simulink model "Sim3_GFo_L_Filter"  (R2018a)
settings: Solver=ode1  StartTime=0.0  StopTime=2.5  FixedStep=Time_Step  MaxStep=1e-4  RelTol=1e-3
undefined symbols (not defined in the file): Lg, Rg, Theta0, Time_Step, Ug, V0, VSC01_id0
libraries: powerlib x43, Control_Lib x9, simulink x8, powerlib_meascontrol x1
(part 2 of 3)

== system Sim3_GFo_L_Filter/VSC_pwm ==
  note: do not modify this part if you use the update loaflow script
  note: Common Inputs
  note: Power part
  note: Measurements and normalization
  note: Control part
  dE_set (pu) : Inport
  dP_set (pu) : Inport  Port=2
  1/Ib2 : Gain  Gain=1/Vb2
  1/Ib3 : Gain  Gain=1/Ib2
  Add : Sum
  Add1 : Sum
  Bridge_Model : Subsystem
  Bus01 : powerlib/Measurements/Three-Phase V-I Measurement  VoltageMeasurement=phase-to-ground  SetLabelV=off  LabelV=Vabc  Vpu=off  VpuLL=off  CurrentMeasurement=yes  SetLabelI=off  LabelI=Iabc  Ipu=off  Pbase=100e6  Vbase=500e3  OutputType=Complex  PhasorSimulation=off  PSBequivalent=0
  Control loops : Subsystem
  DC Voltage Source : powerlib/Electrical Sources/DC Voltage Source  Amplitude=Udcn  Measurements=Voltage
  Memory1 : Memory  InitialCondition=[Va0 Vb0 Vc0]
  Output_Transformer : powerlib/Elements/Three-Phase Transformer (Two Windings)  Winding1Connection=Yg  Winding2Connection=Yg  CoreType=Three single-phase transformers  SetSaturation=off  Hysteresis=off  DataFile='hysteresis'  SetInitialFlux=off  Measurements=None  UNITS=pu  NominalPower=[Sn , fb]  Winding1=[Un1 , Rt_pu/2 , Lt_pu/2]  Winding2=[Un2 , Rt_pu/2 , Lt_pu/2]  Rm=Rm_pu  Lm=Lm_pu  L0=0.5  Saturation=[ 0,0 ; 0.0024,1.2 ; 1.0,1.52 ]  InitialFluxes=[ 0.8 , -0.8 , 0.7 ]  BreakLoop=off  DiscreteSolver=Trapezoidal iterative  DataType=off  TransfoNumber=1
  Pinit : Constant  Value=P0
  Source_For_LF : powerlib/Electrical Sources/Three-Phase Source  Commented=on  InternalConnection=Yg  VoltagePhases=off  Voltage=(400000)*1.00064  PhaseAngle=0.38118  Voltage_phases=[25e3 25e3 25e3]/sqrt(3)  PhaseAngles_phases=[0 -120 +120]  Frequency=fb  NonIdealSource=off  SpecifyImpedance=off  Resistance=0  Inductance=0  ShortCircuitLevel=100e6  BaseVoltage=Un  XRratio=7  BusType=PQ  Pref=P0*Sb  Qref=Q0*Sb  Prefabc=[10e3, 10e3, 10e3]  Qrefabc=[0, 0, 0]  Qmin=-inf  Qmax=inf
  Vvsc_init : Constant  Value=Vvsc0
  mp3 : Gain  Gain=Vb1
  A : PMIOPort  Side=Right
  B : PMIOPort  Port=2  Side=Right
  C : PMIOPort  Port=3  Side=Right
  m : Outport  VectorParamsAs1DForOutWhenUnconnected=off
  wires:
  Add/1 -> Control loops/2(P_set)
  Control loops/2(m) -> m/1  "Control"
  mp3/1 -> Memory1/1
  1/Ib3/1 -> Control loops/4(ig_abc_pu)  "ig_pu"
  1/Ib2/1 -> Control loops/3(vg_abc_pu)  "vg_pu"
  [vg_meas] -> 1/Ib2/1
  Control loops/1(vm_abc_ref_pu) -> mp3/1
  Add1/1 -> Control loops/1(E_set)
  Memory1/1 -> Bridge_Model/1(Uref)
  dP_set (pu)/1 -> Add/1
  Pinit/1 -> Add/2
  Vvsc_init/1 -> Add1/2
  Bus01/1 -> [vg_meas]
  dE_set (pu)/1 -> Add1/1
  Bus01/2 -> [ig_meas]
  [ig_meas] -> 1/Ib3/1
  connections:
  DC Voltage Source/LConn1 -- Bridge_Model/LConn2
  Output_Transformer/RConn1 -- Bus01/LConn1
  Output_Transformer/RConn2 -- Bus01/LConn2
  DC Voltage Source/RConn1 -- Bridge_Model/LConn1
  Output_Transformer/RConn3 -- Bus01/LConn3
  Source_For_LF/RConn2 -- B/RConn1 -- Bus01/RConn2
  Bridge_Model/RConn1 -- Output_Transformer/LConn1
  Bridge_Model/RConn2 -- Output_Transformer/LConn2
  Bridge_Model/RConn3 -- Output_Transformer/LConn3
  Source_For_LF/RConn1 -- A/RConn1 -- Bus01/RConn1
  Source_For_LF/RConn3 -- C/RConn1 -- Bus01/RConn3

== system Sim3_GFo_L_Filter/Infinite_Grid/ pu P//Q computation ==
  v_abc_pu : Inport  PortDimensions=3
  i_abc_pu : Inport  Port=2  PortDimensions=3
  Demux : Demux  Outputs=3
      settings: DisplayOption=none
  Mux : Mux  Inputs=3
  Product1 : Product  InputSameDT=on  SaturateOnIntegerOverflow=on  OutDataTypeStr=Inherit: Same as first input
  Product3 : Product  InputSameDT=on  SaturateOnIntegerOverflow=on  OutDataTypeStr=Inherit: Same as first input
  Sum : Sum  Inputs=+-  InputSameDT=on  SaturateOnIntegerOverflow=on  OutDataTypeStr=Inherit: Same as first input
  Sum1 : Sum  Inputs=1  InputSameDT=on  SaturateOnIntegerOverflow=on  OutDataTypeStr=Inherit: Same as first input
  Sum4 : Sum  Inputs=1  InputSameDT=on  SaturateOnIntegerOverflow=on  OutDataTypeStr=Inherit: Same as first input
  Sum5 : Sum  Inputs=+-  InputSameDT=on  SaturateOnIntegerOverflow=on  OutDataTypeStr=Inherit: Same as first input
  Sum6 : Sum  Inputs=+-  InputSameDT=on  SaturateOnIntegerOverflow=on  OutDataTypeStr=Inherit: Same as first input
  pu->V : Gain  Gain=1/sqrt(3)  SaturateOnIntegerOverflow=on  OutDataTypeStr=Inherit: Same as input  ParamDataTypeStr=Inherit: Same as input
  pu->V1 : Gain  Gain=1/3  SaturateOnIntegerOverflow=on  OutDataTypeStr=Inherit: Same as input  ParamDataTypeStr=Inherit: Same as input
  pu->V2 : Gain  Gain=1/3  SaturateOnIntegerOverflow=on  OutDataTypeStr=Inherit: Same as input  ParamDataTypeStr=Inherit: Same as input
  p_u : Outport  VectorParamsAs1DForOutWhenUnconnected=off
  q_u : Outport  Port=2  VectorParamsAs1DForOutWhenUnconnected=off
  wires:
  pu->V/1 -> pu->V2/1  "Q"
  Mux/1 -> Product3/1
  Sum6/1 -> Mux/2
  Sum5/1 -> Mux/1
  Sum/1 -> Mux/3
  Demux/3 -> Sum6/1, Sum5/2
  Demux/2 -> Sum5/1, Sum/2
  Demux/1 -> Sum6/2, Sum/1
  Sum4/1 -> pu->V1/1
  i_abc_pu/1 -> Product3/2, Product1/2
  v_abc_pu/1 -> Demux/1, Product1/1
  Product1/1 -> Sum4/1
  Product3/1 -> Sum1/1
  Sum1/1 -> pu->V/1
  pu->V1/1 -> p_u/1
  pu->V2/1 -> q_u/1

== system Sim3_GFo_L_Filter/Infinite_Grid/CosSin ==
  Theta_rad : Inport
  Mux : Mux  Inputs=2
  Trigonometric Function : Trigonometry
  Trigonometric Function1 : Trigonometry  Operator=cos
  CosSinTheta : Outport  VectorParamsAs1DForOutWhenUnconnected=off
  wires:
  Trigonometric Function1/1 -> Mux/1
  Mux/1 -> CosSinTheta/1
  Trigonometric Function/1 -> Mux/2
  Theta_rad/1 -> Trigonometric Function1/1, Trigonometric Function/1

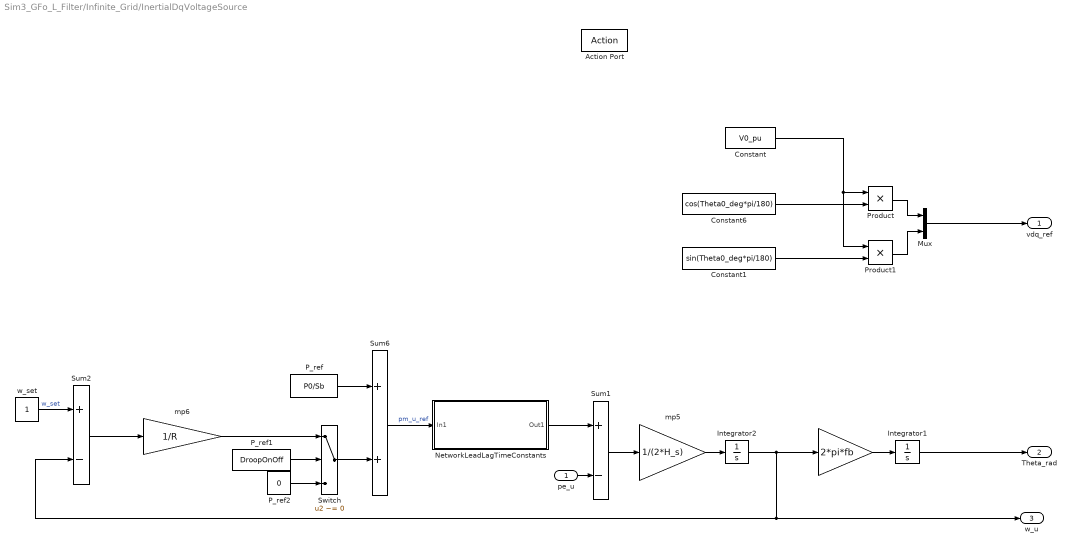
== system Sim3_GFo_L_Filter/Infinite_Grid/InertialDqVoltageSource ==
  pe_u : Inport
  Action Port : ActionPort
  " " : Gain  Gain=2*pi*fb
  Constant : Constant  Value=V0_pu
  Constant1 : Constant  Value=sin(Theta0_deg*pi/180)
  Constant6 : Constant  Value=cos(Theta0_deg*pi/180)
  Integrator1 : Integrator  InitialCondition=Theta0_deg*pi/180
  Integrator2 : Integrator  InitialCondition=1
  Mux : Mux  Inputs=2
  NetworkLeadLagTimeConstants : Subsystem
  P_ref : Constant  Value=P0/Sb
  P_ref1 : Constant  Value=DroopOnOff
  P_ref2 : Constant  Value=0
  Product : Product
  Product1 : Product
  Sum1 : Sum  Inputs=+-
  Sum2 : Sum  Inputs=+-
  Sum6 : Sum
  Switch : Switch  Criteria=u2 ~= 0
  mp5 : Gain  Gain=1/(2*H_s)
  mp6 : Gain  Gain=1/R
  w_set : Constant
  vdq_ref : Outport  VectorParamsAs1DForOutWhenUnconnected=off
  Theta_rad : Outport  Port=2  VectorParamsAs1DForOutWhenUnconnected=off
  w_u : Outport  Port=3  VectorParamsAs1DForOutWhenUnconnected=off
  wires:
  P_ref2/1 -> Switch/3
  mp6/1 -> Switch/1
  Switch/1 -> Sum6/2
  P_ref1/1 -> Switch/2
  NetworkLeadLagTimeConstants/1(Out1) -> Sum1/1
  Mux/1 -> vdq_ref/1
  Product/1 -> Mux/1
  Product1/1 -> Mux/2
  Constant/1 -> Product/1, Product1/1
  Constant6/1 -> Product/2
  Constant1/1 -> Product1/2
  Integrator1/1 -> Theta_rad/1
  w_set/1 -> Sum2/1  "w_set"
  pe_u/1 -> Sum1/2
  " "/1 -> Integrator1/1
  Sum1/1 -> mp5/1
  Sum2/1 -> mp6/1
  P_ref/1 -> Sum6/1
  Integrator2/1 -> " "/1, Sum2/2, w_u/1
  Sum6/1 -> NetworkLeadLagTimeConstants/1(In1)  "pm_u_ref"
  mp5/1 -> Integrator2/1

== system Sim3_GFo_L_Filter/Infinite_Grid/InfiniteDqVoltageSource ==
  Action Port : ActionPort
  Constant : Constant  Value=V0_pu
  Constant1 : Constant  Value=sin(Theta0_deg*pi/180)
  Constant4 : Constant
  Constant6 : Constant  Value=cos(Theta0_deg*pi/180)
  Gain : Gain  Gain=2*pi*fn
  Integrator : Integrator  InitialCondition=Theta0_deg*pi/180
  Mux : Mux  Inputs=2
  Product : Product
  Product1 : Product
  vdq_u_ref : Outport  VectorParamsAs1DForOutWhenUnconnected=off
  Theta_rad : Outport  Port=2  VectorParamsAs1DForOutWhenUnconnected=off
  w_u : Outport  Port=3  VectorParamsAs1DForOutWhenUnconnected=off
  wires:
  Constant4/1 -> Gain/1, w_u/1
  Mux/1 -> vdq_u_ref/1
  Integrator/1 -> Theta_rad/1
  Product1/1 -> Mux/2
  Constant/1 -> Product/1, Product1/1
  Constant6/1 -> Product/2
  Product/1 -> Mux/1
  Gain/1 -> Integrator/1
  Constant1/1 -> Product1/2

== system Sim3_GFo_L_Filter/Infinite_Grid/Source_For_OP ==
  v_abc_ref : Inport
  Controlled Voltage Source1 : powerlib/Electrical Sources/Controlled Voltage Source  Initialize=off  Source_Type=AC  Amplitude=V0*Ub*sqrt(2/3)*sin(Theta0)  Phase=(Theta0*180/pi)  Frequency=fb  Measurements=None
  Controlled Voltage Source2 : powerlib/Electrical Sources/Controlled Voltage Source  Initialize=off  Source_Type=AC  Amplitude=V0*Ub*sqrt(2/3)*sin(Theta0-2*pi/3)  Phase=(Theta0*180/pi)-120  Frequency=fb  Measurements=None
  Controlled Voltage Source3 : powerlib/Electrical Sources/Controlled Voltage Source  Initialize=off  Source_Type=AC  Amplitude=V0*Ub*sqrt(2/3)*sin(Theta0-4*pi/3)  Phase=(Theta0*180/pi)+120  Frequency=fb  Measurements=None
  Demux : Demux  Outputs=3
  Step : Step  Time=1e-9  SampleTime=0
  Subsystem3 : Subsystem
  Three-Phase Source1 : powerlib/Electrical Sources/Three-Phase Source  InternalConnection=Yn  VoltagePhases=off  Voltage=V0_pu*Ub  PhaseAngle=Theta0_deg  Voltage_phases=[25e3 25e3 25e3]/sqrt(3)  PhaseAngles_phases=[0 -120 +120]  Frequency=fb  NonIdealSource=off  SpecifyImpedance=off  Resistance=0.8929  Inductance=16.58e-3  ShortCircuitLevel=100e6  BaseVoltage=25e3  XRratio=7  BusType=swing  Pref=10e3  Qref=0  Prefabc=[10e3, 10e3, 10e3]  Qrefabc=[0, 0, 0]  Qmin=-inf  Qmax=inf
  A : PMIOPort  Side=Right
  B : PMIOPort  Port=2  Side=Right
  C : PMIOPort  Port=3  Side=Right
  N : PMIOPort  Port=4  Side=Left
  wires:
  Step/1 -> Subsystem3/1(switch)
  Demux/3 -> Controlled Voltage Source3/1
  Demux/1 -> Controlled Voltage Source1/1
  v_abc_ref/1 -> Demux/1
  Demux/2 -> Controlled Voltage Source2/1
  connections:
  Three-Phase Source1/RConn3 -- Subsystem3/LConn6
  Three-Phase Source1/RConn2 -- Subsystem3/LConn5
  Three-Phase Source1/RConn1 -- Subsystem3/LConn4
  Controlled Voltage Source3/RConn1 -- Subsystem3/LConn3
  Controlled Voltage Source2/RConn1 -- Subsystem3/LConn2
  Controlled Voltage Source1/RConn1 -- Subsystem3/LConn1
  Subsystem3/RConn3 -- C/RConn1
  Subsystem3/RConn2 -- B/RConn1
  Subsystem3/RConn1 -- A/RConn1
  Controlled Voltage Source1/LConn1 -- Controlled Voltage Source2/LConn1 -- N/RConn1 -- Three-Phase Source1/LConn1 -- Controlled Voltage Source3/LConn1

== system Sim3_GFo_L_Filter/VSC_average/Bridge_Model ==
  Uref : Inport
  Constant : Constant
  Memory : Memory
  NOT1 : Logic  Operator=NOT  IconShape=distinctive  AllPortsSameDT=off  OutDataTypeStr=boolean
  Saturation : Saturate  UpperLimit=1  LowerLimit=-1
  Three-Phase Breaker1 : powerlib/Elements/Three-Phase Breaker  InitialState=closed  SwitchA=on  SwitchB=on  SwitchC=on  SwitchTimes="[4/60  10/60]"  External=on  BreakerResistance=0.001  SnubberResistance=1e6  SnubberCapacitance=inf  Measurements=None
  Three-Phase Breaker2 : powerlib/Elements/Three-Phase Breaker  InitialState=open  SwitchA=on  SwitchB=on  SwitchC=on  SwitchTimes="[4/60  10/60]"  External=on  BreakerResistance=0.001  SnubberResistance=1e6  SnubberCapacitance=inf  Measurements=None
  Three-Phase Source : powerlib/Electrical Sources/Three-Phase Source  InternalConnection=Yg  VoltagePhases=off  Voltage=Vvsc0*Un1  PhaseAngle=Theta_vsc0  Voltage_phases=[25e3 25e3 25e3]/sqrt(3)  PhaseAngles_phases=[0 -120 +120]  Frequency=fb  NonIdealSource=off  SpecifyImpedance=off  Resistance=0  Inductance=0  ShortCircuitLevel=100e6  BaseVoltage=VSC01_Un1  XRratio=7  BusType=swing  Pref=0.3  Qref=0  Prefabc=[10e3, 10e3, 10e3]  Qrefabc=[0, 0, 0]  Qmin=-Inf  Qmax=Inf
  Universal Bridge : powerlib/Power Electronics/Universal Bridge  Arms=3  SnubberResistance=1e5  SnubberCapacitance=inf  Device=Average-model based VSC  Ron=1e-3  Lon=0  ForwardVoltages="[  0  0  ]"  ForwardVoltage=0  GTOparameters=[ 10e-6 , 20e-6 ]  IGBTparameters=[ 1e-6 , 2e-6 ]  Measurements=None  Measurements_2=None  converterType=Rectifier
  mp3 : Gain  Gain=2/Udcn
  PhA : PMIOPort  Side=Right
  PhB : PMIOPort  Port=2  Side=Right
  PhC : PMIOPort  Port=3  Side=Right
  Vdc+ : PMIOPort  Port=4  Side=Left
  Vdc- : PMIOPort  Port=5  Side=Left
  wires:
  Saturation/1 -> Universal Bridge/1
  Constant/1 -> Memory/1
  NOT1/1 -> Three-Phase Breaker1/1
  Memory/1 -> NOT1/1, Three-Phase Breaker2/1
  mp3/1 -> Saturation/1
  Uref/1 -> mp3/1
  connections:
  Three-Phase Breaker2/LConn1 -- Three-Phase Breaker1/LConn1 -- PhA/RConn1
  Three-Phase Breaker2/LConn2 -- Three-Phase Breaker1/LConn2 -- PhB/RConn1
  Three-Phase Breaker2/LConn3 -- Three-Phase Breaker1/LConn3 -- PhC/RConn1
  Three-Phase Breaker2/RConn1 -- Universal Bridge/LConn1
  Three-Phase Breaker2/RConn2 -- Universal Bridge/LConn2
  Three-Phase Breaker2/RConn3 -- Universal Bridge/LConn3
  Three-Phase Source/RConn1 -- Three-Phase Breaker1/RConn1
  Three-Phase Source/RConn2 -- Three-Phase Breaker1/RConn2
  Three-Phase Source/RConn3 -- Three-Phase Breaker1/RConn3
  Universal Bridge/RConn1 -- Vdc+/RConn1
  Universal Bridge/RConn2 -- Vdc-/RConn1

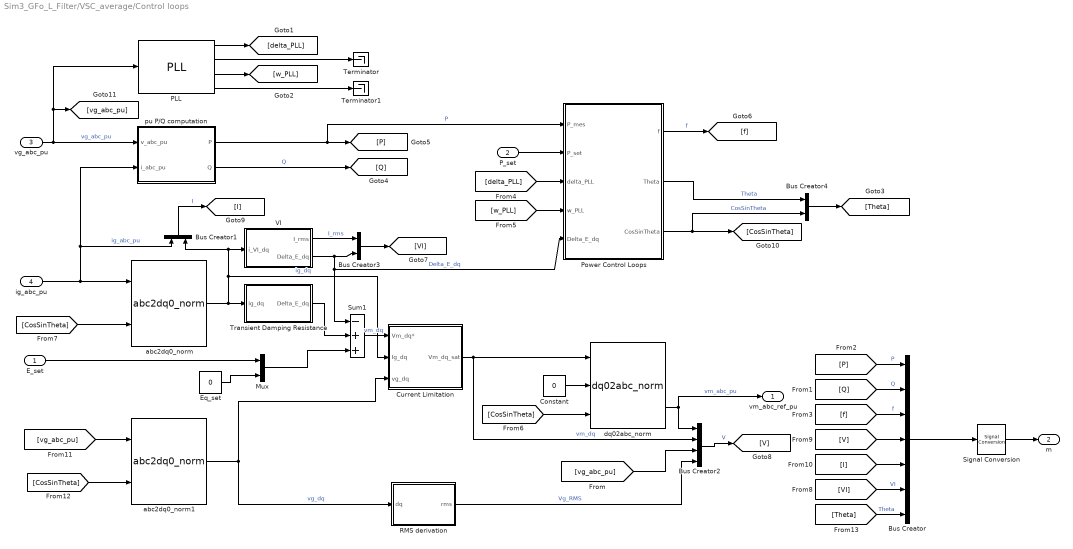
== system Sim3_GFo_L_Filter/VSC_average/Control loops ==
  E_set : Inport
  P_set : Inport  Port=2
  vg_abc_pu : Inport  Port=3
  ig_abc_pu : Inport  Port=4
  " pu P/Q computation" : Subsystem  DialogController=POWERSYS.PowerSysDialog
  Bus Creator : BusCreator  Inputs=7
  Bus Creator1 : BusCreator  Inputs=2
  Bus Creator2 : BusCreator  Inputs=4
  Bus Creator3 : BusCreator  Inputs=2
  Bus Creator4 : BusCreator  Inputs=2
  Constant : Constant  Value=0
  Current Limitation : Subsystem
  Eq_set : Constant  Value=0
  Mux : Mux  Inputs=2
  PLL : Control_Lib/PLL  fb=fb  Tr_PLL=Tr_PLL  Theta0=Theta0
      settings: SourceProductName=VSC_Lib
  Power Control Loops : Subsystem
  RMS derivation : Subsystem
  Signal Conversion : SignalConversion  OverrideOpt=off
  Sum1 : Sum  Inputs=-++
  Terminator : Terminator
  Terminator1 : Terminator
  Transient Damping Resistance : Subsystem
  VI : Subsystem
  abc2dq0_norm : Control_Lib/abc2dq0_norm  referenceAxisMode=Reference axis at 90 degrees behind phase_a  baseUpdateGain=1/sqrt(3)
      settings: SourceProductName=VSC_Lib
  abc2dq0_norm1 : Control_Lib/abc2dq0_norm  referenceAxisMode=Reference axis at 90 degrees behind phase_a  baseUpdateGain=1/sqrt(3)
      settings: SourceProductName=VSC_Lib
  dq02abc_norm : Control_Lib/dq02abc_norm  referenceAxisMode=Reference axis at 90 degrees behind phase_a  baseUpdateGain=sqrt(3)
      settings: SourceProductName=VSC_Lib
  vm_abc_ref_pu : Outport  VectorParamsAs1DForOutWhenUnconnected=off
  m : Outport  Port=2  VectorParamsAs1DForOutWhenUnconnected=off
  wires:
  [Theta] -> Bus Creator/7  "Theta"
  Bus Creator4/1 -> [Theta]
  RMS derivation/1(rms) -> Bus Creator2/4  "Vg_RMS"
  [vg_abc_pu] -> Bus Creator2/3
  Bus Creator3/1 -> [VI]
  PLL/4 -> Terminator1/1
  PLL/2 -> Terminator/1
  PLL/1 -> [delta_PLL]
  Constant/1 -> dq02abc_norm/2
  Power Control Loops/3(CosSinTheta) -> [CosSinTheta], Bus Creator4/2  "CosSinTheta"
  PLL/3 -> [w_PLL]
  [I] -> Bus Creator/5
  Bus Creator1/1 -> [I]  "I"
  Bus Creator/1 -> Signal Conversion/1
  [VI] -> Bus Creator/6  "VI"
  [V] -> Bus Creator/4
  Bus Creator2/1 -> [V]  "V"
  Eq_set/1 -> Mux/2
  Mux/1 -> Sum1/3
  VI/1(I_rms) -> Bus Creator3/1  "I_rms"
  Transient Damping Resistance/1("Delta_E_dq ") -> Sum1/2
  VI/2(Delta_E_dq) -> Bus Creator3/2, Sum1/1, Power Control Loops/5(Delta_E_dq)  "Delta_E_dq"
  [CosSinTheta] -> abc2dq0_norm/2
  [CosSinTheta] -> dq02abc_norm/3
  Power Control Loops/2(Theta) -> Bus Creator4/1  "Theta"
  abc2dq0_norm/2 -> Bus Creator1/2, VI/1(i_VI_dq), Current Limitation/2(Ig_dq), Transient Damping Resistance/1(ig_dq)  "ig_dq"
  ig_abc_pu/1 -> abc2dq0_norm/1, " pu P/Q computation"/2(i_abc_pu), Bus Creator1/1  "ig_abc_pu"
  " pu P/Q computation"/1(P) -> [P], Power Control Loops/1(P_mes)  "P"
  vg_abc_pu/1 -> PLL/1, [vg_abc_pu], " pu P/Q computation"/1(v_abc_pu)  "vg_abc_pu"
  Power Control Loops/1(f) -> [f]  "f"
  [w_PLL] -> Power Control Loops/4(w_PLL)
  P_set/1 -> Power Control Loops/2(P_set)
  [delta_PLL] -> Power Control Loops/3(delta_PLL)
  Current Limitation/1(Vm_dq_sat) -> dq02abc_norm/1, Bus Creator2/2  "vm_dq"
  " pu P/Q computation"/2(Q) -> [Q]  "Q"
  E_set/1 -> Mux/1
  dq02abc_norm/2 -> Bus Creator2/1, vm_abc_ref_pu/1  "vm_abc_pu"
  [f] -> Bus Creator/3  "f"
  [Q] -> Bus Creator/2  "Q"
  [P] -> Bus Creator/1  "P"
  Signal Conversion/1 -> m/1
  Sum1/1 -> Current Limitation/1(Vm_dq*)  "vm_dq"
  [vg_abc_pu] -> abc2dq0_norm1/1
  [CosSinTheta] -> abc2dq0_norm1/2
  abc2dq0_norm1/2 -> Current Limitation/3(vg_dq), RMS derivation/1(dq)  "vg_dq"

== system Sim3_GFo_L_Filter/VSC_pwm/Bridge_Model ==
  Uref : Inport
  Constant : Constant
  Detailed : Subsystem
  Memory : Memory
  NOT1 : Logic  Operator=NOT  IconShape=distinctive  AllPortsSameDT=off  OutDataTypeStr=boolean
  Saturation : Saturate  UpperLimit=1  LowerLimit=-1
  Three-Phase Breaker1 : powerlib/Elements/Three-Phase Breaker  InitialState=closed  SwitchA=on  SwitchB=on  SwitchC=on  SwitchTimes="[4/60  10/60]"  External=on  BreakerResistance=0.001  SnubberResistance=1e6  SnubberCapacitance=inf  Measurements=None
  Three-Phase Breaker2 : powerlib/Elements/Three-Phase Breaker  InitialState=open  SwitchA=on  SwitchB=on  SwitchC=on  SwitchTimes="[4/60  10/60]"  External=on  BreakerResistance=0.001  SnubberResistance=1e6  SnubberCapacitance=inf  Measurements=None
  Three-Phase Source : powerlib/Electrical Sources/Three-Phase Source  InternalConnection=Yg  VoltagePhases=off  Voltage=Vvsc0*Un1  PhaseAngle=Theta_vsc0  Voltage_phases=[25e3 25e3 25e3]/sqrt(3)  PhaseAngles_phases=[0 -120 +120]  Frequency=fb  NonIdealSource=off  SpecifyImpedance=off  Resistance=0  Inductance=0  ShortCircuitLevel=100e6  BaseVoltage=VSC01_Un1  XRratio=7  BusType=swing  Pref=0.3  Qref=0  Prefabc=[10e3, 10e3, 10e3]  Qrefabc=[0, 0, 0]  Qmin=-Inf  Qmax=Inf
  mp3 : Gain  Gain=2/Udcn
  PhA : PMIOPort  Side=Right
  PhB : PMIOPort  Port=2  Side=Right
  PhC : PMIOPort  Port=3  Side=Right
  Vdc+ : PMIOPort  Port=4  Side=Left
  Vdc- : PMIOPort  Port=5  Side=Left
  wires:
  Saturation/1 -> Detailed/1(Urref)
  Constant/1 -> Memory/1
  NOT1/1 -> Three-Phase Breaker1/1
  Memory/1 -> NOT1/1, Three-Phase Breaker2/1
  mp3/1 -> Saturation/1
  Uref/1 -> mp3/1
  connections:
  Three-Phase Breaker2/LConn1 -- Three-Phase Breaker1/LConn1 -- PhA/RConn1
  Three-Phase Breaker2/LConn2 -- Three-Phase Breaker1/LConn2 -- PhB/RConn1
  Three-Phase Breaker2/LConn3 -- Three-Phase Breaker1/LConn3 -- PhC/RConn1
  Detailed/LConn1 -- Three-Phase Breaker2/RConn1
  Detailed/LConn2 -- Three-Phase Breaker2/RConn2
  Detailed/LConn3 -- Three-Phase Breaker2/RConn3
  Three-Phase Source/RConn1 -- Three-Phase Breaker1/RConn1
  Three-Phase Source/RConn2 -- Three-Phase Breaker1/RConn2
  Three-Phase Source/RConn3 -- Three-Phase Breaker1/RConn3
  Detailed/RConn1 -- Vdc+/RConn1
  Detailed/RConn2 -- Vdc-/RConn1

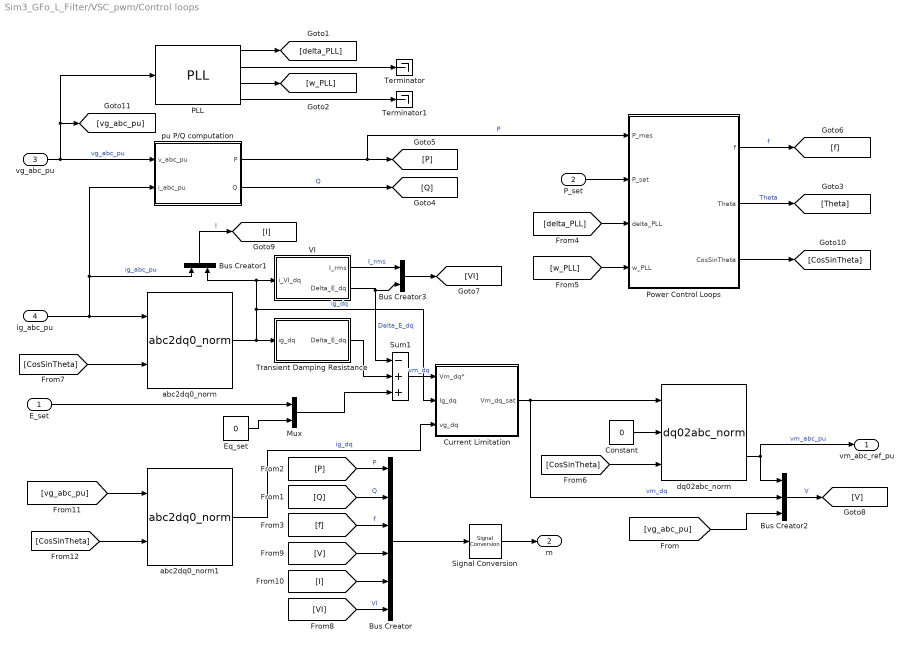
== system Sim3_GFo_L_Filter/VSC_pwm/Control loops ==
  E_set : Inport
  P_set : Inport  Port=2
  vg_abc_pu : Inport  Port=3
  ig_abc_pu : Inport  Port=4
  " pu P/Q computation" : Subsystem  DialogController=POWERSYS.PowerSysDialog
  Bus Creator : BusCreator  Inputs=6
  Bus Creator1 : BusCreator  Inputs=2
  Bus Creator2 : BusCreator  Inputs=3
  Bus Creator3 : BusCreator  Inputs=2
  Constant : Constant  Value=0
  Current Limitation : Subsystem
  Eq_set : Constant  Value=0
  Mux : Mux  Inputs=2
  PLL : Control_Lib/PLL  fb=fb  Tr_PLL=Tr_PLL  Theta0=Theta0
      settings: SourceProductName=VSC_Lib
  Power Control Loops : Subsystem
  Signal Conversion : SignalConversion  OverrideOpt=off
  Sum1 : Sum  Inputs=-++
  Terminator : Terminator
  Terminator1 : Terminator
  Transient Damping Resistance : Subsystem
  VI : Subsystem
  abc2dq0_norm : Control_Lib/abc2dq0_norm  referenceAxisMode=Reference axis at 90 degrees behind phase_a  baseUpdateGain=1/sqrt(3)
      settings: SourceProductName=VSC_Lib
  abc2dq0_norm1 : Control_Lib/abc2dq0_norm  referenceAxisMode=Reference axis at 90 degrees behind phase_a  baseUpdateGain=1/sqrt(3)
      settings: SourceProductName=VSC_Lib
  dq02abc_norm : Control_Lib/dq02abc_norm  referenceAxisMode=Reference axis at 90 degrees behind phase_a  baseUpdateGain=sqrt(3)
      settings: SourceProductName=VSC_Lib
  vm_abc_ref_pu : Outport  VectorParamsAs1DForOutWhenUnconnected=off
  m : Outport  Port=2  VectorParamsAs1DForOutWhenUnconnected=off
  wires:
  [vg_abc_pu] -> Bus Creator2/3
  Bus Creator3/1 -> [VI]
  PLL/4 -> Terminator1/1
  PLL/2 -> Terminator/1
  PLL/1 -> [delta_PLL]
  Constant/1 -> dq02abc_norm/2
  Power Control Loops/3(CosSinTheta) -> [CosSinTheta]
  PLL/3 -> [w_PLL]
  [I] -> Bus Creator/5
  Bus Creator1/1 -> [I]  "I"
  Bus Creator/1 -> Signal Conversion/1
  [VI] -> Bus Creator/6  "VI"
  [V] -> Bus Creator/4
  Bus Creator2/1 -> [V]  "V"
  Eq_set/1 -> Mux/2
  Mux/1 -> Sum1/3
  VI/1(I_rms) -> Bus Creator3/1  "I_rms"
  Transient Damping Resistance/1("Delta_E_dq ") -> Sum1/2
  VI/2(Delta_E_dq) -> Sum1/1, Bus Creator3/2  "Delta_E_dq"
  [CosSinTheta] -> abc2dq0_norm/2
  [CosSinTheta] -> dq02abc_norm/3
  Power Control Loops/2(Theta) -> [Theta]  "Theta"
  abc2dq0_norm/2 -> Bus Creator1/2, VI/1(i_VI_dq), Current Limitation/2(Ig_dq), Transient Damping Resistance/1(ig_dq)  "ig_dq"
  ig_abc_pu/1 -> abc2dq0_norm/1, " pu P/Q computation"/2(i_abc_pu), Bus Creator1/1  "ig_abc_pu"
  " pu P/Q computation"/1(P) -> [P], Power Control Loops/1(P_mes)  "P"
  vg_abc_pu/1 -> PLL/1, [vg_abc_pu], " pu P/Q computation"/1(v_abc_pu)  "vg_abc_pu"
  Power Control Loops/1(f) -> [f]  "f"
  [w_PLL] -> Power Control Loops/4(w_PLL)
  P_set/1 -> Power Control Loops/2(P_set)
  [delta_PLL] -> Power Control Loops/3(delta_PLL)
  Current Limitation/1(Vm_dq_sat) -> dq02abc_norm/1, Bus Creator2/2  "vm_dq"
  " pu P/Q computation"/2(Q) -> [Q]  "Q"
  E_set/1 -> Mux/1
  dq02abc_norm/2 -> Bus Creator2/1, vm_abc_ref_pu/1  "vm_abc_pu"
  [f] -> Bus Creator/3  "f"
  [Q] -> Bus Creator/2  "Q"
  [P] -> Bus Creator/1  "P"
  Signal Conversion/1 -> m/1
  Sum1/1 -> Current Limitation/1(Vm_dq*)  "vm_dq"
  [vg_abc_pu] -> abc2dq0_norm1/1
  [CosSinTheta] -> abc2dq0_norm1/2
  abc2dq0_norm1/2 -> Current Limitation/3(vg_dq)  "ig_dq"

== system Sim3_GFo_L_Filter/Infinite_Grid/InertialDqVoltageSource/NetworkLeadLagTimeConstants ==
  In1 : Inport
  Integrator3 : Integrator  InitialCondition=(P0/Sb)*(1-TN/TD)
  Sum1 : Sum
  Sum2 : Sum  Inputs=+-
  mp1 : Gain  Gain=TN/TD
  mp2 : Gain  Gain=1-TN/TD
  mp3 : Gain  Gain=1/TD
  Out1 : Outport  VectorParamsAs1DForOutWhenUnconnected=off
  wires:
  Sum2/1 -> mp3/1
  mp3/1 -> Integrator3/1
  Integrator3/1 -> Sum1/2, Sum2/2
  In1/1 -> mp1/1, mp2/1
  mp2/1 -> Sum2/1
  mp1/1 -> Sum1/1
  Sum1/1 -> Out1/1

== system Sim3_GFo_L_Filter/Infinite_Grid/Source_For_OP/Subsystem3 ==
  switch : Inport
  Breaker : powerlib/Elements/Breaker  InitialState=0  SwitchingTimes="[1/60  5/60]"  External=on  BreakerResistance=0.001  SnubberResistance=1e6  SnubberCapacitance=inf  Measurements=None  MoreParameters=on  NoBreakLoop=off
  Breaker1 : powerlib/Elements/Breaker  InitialState=0  SwitchingTimes="[1/60  5/60]"  External=on  BreakerResistance=0.001  SnubberResistance=1e6  SnubberCapacitance=inf  Measurements=None  MoreParameters=on  NoBreakLoop=off
  Breaker2 : powerlib/Elements/Breaker  InitialState=0  SwitchingTimes="[1/60  5/60]"  External=on  BreakerResistance=0.001  SnubberResistance=1e6  SnubberCapacitance=inf  Measurements=None  MoreParameters=on  NoBreakLoop=off
  Breaker3 : powerlib/Elements/Breaker  InitialState=1  SwitchingTimes="[1/60  5/60]"  External=on  BreakerResistance=0.001  SnubberResistance=1e6  SnubberCapacitance=inf  Measurements=None  MoreParameters=on  NoBreakLoop=off
  Breaker4 : powerlib/Elements/Breaker  InitialState=1  SwitchingTimes="[1/60  5/60]"  External=on  BreakerResistance=0.001  SnubberResistance=1e6  SnubberCapacitance=inf  Measurements=None  MoreParameters=on  NoBreakLoop=off
  Breaker5 : powerlib/Elements/Breaker  InitialState=1  SwitchingTimes="[1/60  5/60]"  External=on  BreakerResistance=0.001  SnubberResistance=1e6  SnubberCapacitance=inf  Measurements=None  MoreParameters=on  NoBreakLoop=off
  Logical Operator : Logic  Operator=NOT  AllPortsSameDT=off  OutDataTypeStr=boolean
  A : PMIOPort  Side=Left
  B : PMIOPort  Port=2  Side=Left
  C : PMIOPort  Port=3  Side=Left
  Ainit : PMIOPort  Port=4  Side=Left
  Binit : PMIOPort  Port=5  Side=Left
  Cinit : PMIOPort  Port=6  Side=Left
  a : PMIOPort  Port=7  Side=Right
  b : PMIOPort  Port=8  Side=Right
  c : PMIOPort  Port=9  Side=Right
  wires:
  Logical Operator/1 -> Breaker3/1, Breaker4/1, Breaker5/1
  switch/1 -> Logical Operator/1, Breaker/1, Breaker1/1, Breaker2/1
  connections:
  Breaker4/RConn1 -- Breaker1/RConn1 -- b/RConn1
  a/RConn1 -- Breaker3/RConn1 -- Breaker/RConn1
  Breaker1/LConn1 -- B/RConn1
  Breaker3/LConn1 -- Ainit/RConn1
  Breaker2/LConn1 -- C/RConn1
  Breaker4/LConn1 -- Binit/RConn1
  Breaker2/RConn1 -- Breaker5/RConn1 -- c/RConn1
  Breaker5/LConn1 -- Cinit/RConn1
  Breaker/LConn1 -- A/RConn1

== system Sim3_GFo_L_Filter/VSC_average/Control loops/ pu P//Q computation ==
  v_abc_pu : Inport  PortDimensions=3
  i_abc_pu : Inport  Port=2  PortDimensions=3
  Demux : Demux  Outputs=3
      settings: DisplayOption=none
  Mux : Mux  Inputs=3
  Product1 : Product  InputSameDT=on  SaturateOnIntegerOverflow=on  OutDataTypeStr=Inherit: Same as first input
  Product3 : Product  InputSameDT=on  SaturateOnIntegerOverflow=on  OutDataTypeStr=Inherit: Same as first input
  Sum : Sum  Inputs=+-  InputSameDT=on  SaturateOnIntegerOverflow=on  OutDataTypeStr=Inherit: Same as first input
  Sum1 : Sum  Inputs=1  InputSameDT=on  SaturateOnIntegerOverflow=on  OutDataTypeStr=Inherit: Same as first input
  Sum4 : Sum  Inputs=1  InputSameDT=on  SaturateOnIntegerOverflow=on  OutDataTypeStr=Inherit: Same as first input
  Sum5 : Sum  Inputs=+-  InputSameDT=on  SaturateOnIntegerOverflow=on  OutDataTypeStr=Inherit: Same as first input
  Sum6 : Sum  Inputs=+-  InputSameDT=on  SaturateOnIntegerOverflow=on  OutDataTypeStr=Inherit: Same as first input
  pu->V : Gain  Gain=1/sqrt(3)  SaturateOnIntegerOverflow=on  OutDataTypeStr=Inherit: Same as input  ParamDataTypeStr=Inherit: Same as input
  pu->V1 : Gain  Gain=1/3  SaturateOnIntegerOverflow=on  OutDataTypeStr=Inherit: Same as input  ParamDataTypeStr=Inherit: Same as input
  pu->V2 : Gain  Gain=1/3  SaturateOnIntegerOverflow=on  OutDataTypeStr=Inherit: Same as input  ParamDataTypeStr=Inherit: Same as input
  P : Outport  VectorParamsAs1DForOutWhenUnconnected=off
  Q : Outport  Port=2  VectorParamsAs1DForOutWhenUnconnected=off
  wires:
  pu->V2/1 -> Q/1
  pu->V1/1 -> P/1
  Sum1/1 -> pu->V/1
  Product3/1 -> Sum1/1
  Product1/1 -> Sum4/1
  v_abc_pu/1 -> Product1/1, Demux/1
  i_abc_pu/1 -> Product1/2, Product3/2
  Sum4/1 -> pu->V1/1
  Demux/1 -> Sum/1, Sum6/2
  Demux/2 -> Sum/2, Sum5/1
  Demux/3 -> Sum5/2, Sum6/1
  Sum/1 -> Mux/3
  Sum5/1 -> Mux/1
  Sum6/1 -> Mux/2
  Mux/1 -> Product3/1
  pu->V/1 -> pu->V2/1  "Q"

== system Sim3_GFo_L_Filter/VSC_average/Control loops/Current Limitation ==
  note: Current limitation
  Vm_dq* : Inport
  Ig_dq : Inport  Port=2
  vg_dq : Inport  Port=3
  Constant : Constant  Value=I_max_pu
  Current control : Subsystem
  Demux : Demux  Outputs=2
  Demux2 : Demux  Outputs=2
  Inverse Current control : Subsystem
  Mux : Mux  Inputs=2
  Product{,1..3} (4 alike) : Product
  Saturation Dynamic : simulink/Discontinuities/Saturation Dynamic  OutMin=[]  OutMax=[]  OutDataTypeStr=Inherit: Same as second input  OutDataType=fixdt(1, 16)  OutScaling=2^-10  DoSatur=off
  Sqrt : Sqrt  SaturateOnIntegerOverflow=on
  Sum : Sum
  Trigonometric Function : Trigonometry  Operator=atan2  NumberOfIterations=5  OutputSignalType=real
  Trigonometric Function1 : Trigonometry  Operator=cos
  Trigonometric Function2 : Trigonometry
  w_set1 : Constant
  w_set2 : Constant
  w_set3 : Constant  Value=0
  Vm_dq_sat : Outport  VectorParamsAs1DForOutWhenUnconnected=off
  wires:
  w_set3/1 -> Saturation Dynamic/3
  Constant/1 -> Saturation Dynamic/1
  Mux/1 -> Current control/1(Ig_dq0*)
  Product/1 -> Mux/1
  Demux/1 -> Product1/1, Product1/2
  Demux/2 -> Product2/1, Product2/2
  Trigonometric Function2/1 -> Product3/2
  Product2/1 -> Sum/2
  Trigonometric Function1/1 -> Product/2
  Demux2/1 -> Trigonometric Function/2
  Trigonometric Function/1 -> Trigonometric Function2/1, Trigonometric Function1/1
  Saturation Dynamic/1 -> Product/1, Product3/1
  Product1/1 -> Sum/1
  Sqrt/1 -> Saturation Dynamic/2
  Demux2/2 -> Trigonometric Function/1
  Inverse Current control/1(Is_dq*) -> Demux2/1, Demux/1
  Sum/1 -> Sqrt/1
  Product3/1 -> Mux/2
  Ig_dq/1 -> Inverse Current control/2(Ig_dq), Current control/2(Ig_dq0)
  w_set1/1 -> Inverse Current control/4(w)
  w_set2/1 -> Current control/4(w)
  vg_dq/1 -> Current control/3(vg_dq0), Inverse Current control/3(vg_dq)
  Vm_dq*/1 -> Inverse Current control/1(Vm_dq*)
  Current control/1(vm) -> Vm_dq_sat/1

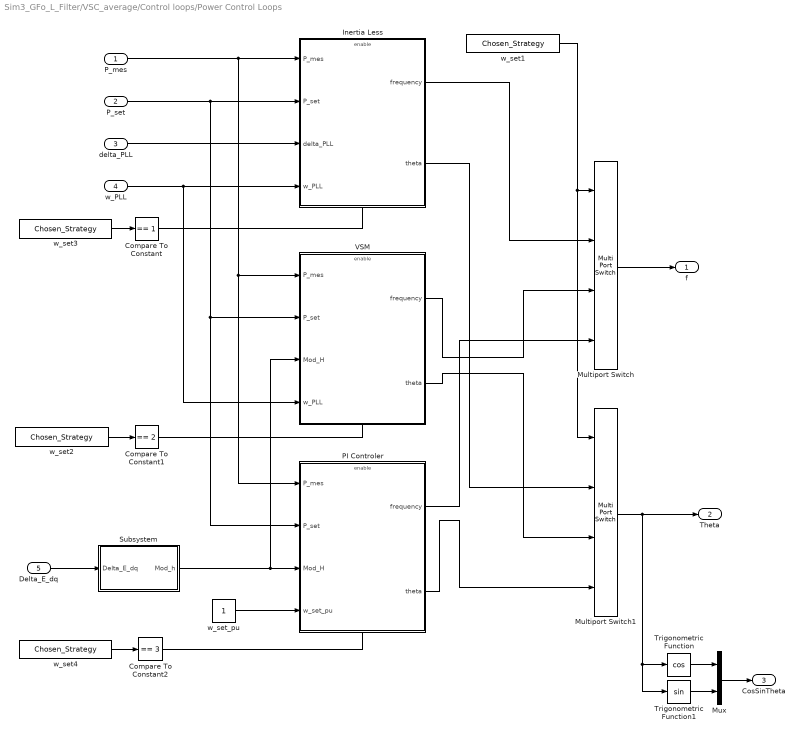
== system Sim3_GFo_L_Filter/VSC_average/Control loops/Power Control Loops ==
  P_mes : Inport
  P_set : Inport  Port=2
  delta_PLL : Inport  Port=3
  w_PLL : Inport  Port=4
  Delta_E_dq : Inport  Port=5
  Compare To Constant : simulink/Logic and Bit Operations/Compare To Constant  relop===  const=1  OutDataTypeStr=boolean
  Compare To Constant1 : simulink/Logic and Bit Operations/Compare To Constant  relop===  const=2  OutDataTypeStr=boolean
  Compare To Constant2 : simulink/Logic and Bit Operations/Compare To Constant  relop===  const=3  OutDataTypeStr=boolean
  Inertia Less : Subsystem
  Multiport Switch : MultiPortSwitch
  Multiport Switch1 : MultiPortSwitch
  Mux : Mux  Inputs=[1 1]
  PI Controler : Subsystem
  Subsystem : Subsystem
  Trigonometric Function : Trigonometry  Operator=cos
  Trigonometric Function1 : Trigonometry
  VSM : Subsystem
  w_set{1..4} (4 alike) : Constant  Value=Chosen_Strategy
  w_set_pu : Constant
  f : Outport  PortDimensions=1  VectorParamsAs1DForOutWhenUnconnected=off
  Theta : Outport  Port=2  VectorParamsAs1DForOutWhenUnconnected=off
  CosSinTheta : Outport  Port=3  PortDimensions=2  VectorParamsAs1DForOutWhenUnconnected=off
  wires:
  Subsystem/1(Mod_h) -> PI Controler/3(Mod_H), VSM/3(Mod_H)
  Delta_E_dq/1 -> Subsystem/1(Delta_E_dq)
  Multiport Switch1/1 -> Trigonometric Function1/1, Trigonometric Function/1, Theta/1
  Trigonometric Function1/1 -> Mux/2
  Mux/1 -> CosSinTheta/1
  Trigonometric Function/1 -> Mux/1
  Compare To Constant2/1 -> PI Controler/Enable
  Compare To Constant1/1 -> VSM/Enable
  Compare To Constant/1 -> Inertia Less/Enable
  w_set4/1 -> Compare To Constant2/1
  w_set2/1 -> Compare To Constant1/1
  w_set3/1 -> Compare To Constant/1
  Inertia Less/1(frequency) -> Multiport Switch/2
  Multiport Switch/1 -> f/1
  Inertia Less/2(theta) -> Multiport Switch1/2
  VSM/2(theta) -> Multiport Switch1/3
  w_set1/1 -> Multiport Switch/1, Multiport Switch1/1
  VSM/1(frequency) -> Multiport Switch/3
  PI Controler/1(frequency) -> Multiport Switch/4
  PI Controler/2(theta) -> Multiport Switch1/4
  w_set_pu/1 -> PI Controler/4(w_set_pu)
  w_PLL/1 -> Inertia Less/4(w_PLL), VSM/4(w_PLL)
  delta_PLL/1 -> Inertia Less/3(delta_PLL)
  P_set/1 -> Inertia Less/2(P_set), VSM/2(P_set), PI Controler/2(P_set)
  P_mes/1 -> Inertia Less/1(P_mes), VSM/1(P_mes), PI Controler/1(P_mes)

== system Sim3_GFo_L_Filter/VSC_average/Control loops/RMS derivation ==
  dq : Inport
  Demux : Demux  Outputs=2
  Sqrt : Sqrt  SaturateOnIntegerOverflow=on
  Square : Math  Operator=square  SaturateOnIntegerOverflow=on
  Square1 : Math  Operator=square  SaturateOnIntegerOverflow=on
  Sum : Sum
  rms : Outport
  wires:
  dq/1 -> Demux/1
  Demux/2 -> Square1/1
  Square/1 -> Sum/1
  Demux/1 -> Square/1
  Sqrt/1 -> rms/1
  Sum/1 -> Sqrt/1
  Square1/1 -> Sum/2

== system Sim3_GFo_L_Filter/VSC_average/Control loops/Transient Damping Resistance ==
  ig_dq : Inport
  Filter w_LF : Subsystem
      mask Display: disp('\omega_{LF} / (s + \omega_{LF})','texmode','on')
  Sum5 : Sum  Inputs=|+-
  nq1 : Gain  Gain=Rv
  "Delta_E_dq " : Outport  VectorParamsAs1DForOutWhenUnconnected=off
  wires:
  nq1/1 -> Filter w_LF/1(e), Sum5/2
  Filter w_LF/1(s) -> Sum5/1
  Sum5/1 -> "Delta_E_dq "/1
  ig_dq/1 -> nq1/1

== system Sim3_GFo_L_Filter/VSC_average/Control loops/VI ==
  note: VI triggering and threshold computation
  note: VI
  i_VI_dq : Inport
  Demux1 : Demux  Outputs=2
      settings: DisplayOption=none
  Gain5 : Gain  Gain=DX_DR
  Gain6 : Gain  Gain=Kp_Rvi_pu
  Gain9 : Gain  Gain=DX_DR
  I_thresh : Constant
  Mux2 : Mux  Inputs=2
  Saturation : Saturate  UpperLimit=I_max_VI_pu-1  LowerLimit=0
  Sum1 : Sum  Inputs=-+|
  Sum7 : Sum  Inputs=|+-
  Sum8 : Sum  Inputs=++|
  dq to phasor : Subsystem
  product{,1..3} (4 alike) : Product  InputSameDT=on  RndMeth=Zero  SaturateOnIntegerOverflow=on  OutDataTypeStr=Inherit: Same as first input
  I_rms : Outport  VectorParamsAs1DForOutWhenUnconnected=off
  Delta_E_dq : Outport  Port=2  VectorParamsAs1DForOutWhenUnconnected=off
  wires:
  Sum1/1 -> Saturation/1
  dq to phasor/1(rms) -> Sum1/2, I_rms/1  "I_rms"
  Saturation/1 -> Gain6/1
  I_thresh/1 -> Sum1/1
  Mux2/1 -> Delta_E_dq/1
  Gain6/1 -> product3/2, product/1, product1/2, product2/2
  product3/1 -> Gain5/1
  product/1 -> Gain9/1
  Demux1/1 -> product1/1, product/2  "igd"
  Demux1/2 -> product2/1, product3/1  "igq"
  product1/1 -> Sum7/1
  Gain5/1 -> Sum7/2
  Gain9/1 -> Sum8/1
  product2/1 -> Sum8/2
  Sum7/1 -> Mux2/1
  Sum8/1 -> Mux2/2
  i_VI_dq/1 -> dq to phasor/1(dq_mes), Demux1/1

== system Sim3_GFo_L_Filter/VSC_pwm/Bridge_Model/Detailed ==
  Urref : Inport
  PWM Generator (2-Level) : powerlib_meascontrol/Pulse & Signal Generators/PWM Generator (2-Level)  ModulatorType=Three-phase bridge (6 pulses)  ModulatorMode=Unsynchronized  Fc=fpwm  Pc=90  nF=27  MinMax="[ -1  1 ]"  SamplingTechnique=Natural  ModulatingSignals=off  m=0.8  Freq=60  Phase=0  Ts=Time_Step  ShowCarrierOutport=off
  Universal Bridge1 : powerlib/Power Electronics/Universal Bridge  Arms=3  SnubberResistance=1e5  SnubberCapacitance=inf  Device=IGBT / Diodes  Ron=1e-3  Lon=0  ForwardVoltages="[  0  0  ]"  ForwardVoltage=0  GTOparameters=[ 10e-6 , 20e-6 ]  IGBTparameters=[ 1e-6 , 2e-6 ]  Measurements=None  Measurements_2=None  converterType=Rectifier
  + : PMIOPort  Side=Right
  A : PMIOPort  Port=2  Side=Left
  B : PMIOPort  Port=3  Side=Left
  - : PMIOPort  Port=4  Side=Right
  C : PMIOPort  Port=5  Side=Left
  wires:
  Urref/1 -> PWM Generator (2-Level)/1
  PWM Generator (2-Level)/1 -> Universal Bridge1/1
  connections:
  Universal Bridge1/RConn1 -- +/RConn1
  Universal Bridge1/RConn2 -- -/RConn1
  Universal Bridge1/LConn2 -- B/RConn1
  Universal Bridge1/LConn1 -- A/RConn1
  Universal Bridge1/LConn3 -- C/RConn1

== system Sim3_GFo_L_Filter/VSC_pwm/Control loops/ pu P//Q computation ==
  v_abc_pu : Inport  PortDimensions=3
  i_abc_pu : Inport  Port=2  PortDimensions=3
  Demux : Demux  Outputs=3
      settings: DisplayOption=none
  Mux : Mux  Inputs=3
  Product1 : Product  InputSameDT=on  SaturateOnIntegerOverflow=on  OutDataTypeStr=Inherit: Same as first input
  Product3 : Product  InputSameDT=on  SaturateOnIntegerOverflow=on  OutDataTypeStr=Inherit: Same as first input
  Sum : Sum  Inputs=+-  InputSameDT=on  SaturateOnIntegerOverflow=on  OutDataTypeStr=Inherit: Same as first input
  Sum1 : Sum  Inputs=1  InputSameDT=on  SaturateOnIntegerOverflow=on  OutDataTypeStr=Inherit: Same as first input
  Sum4 : Sum  Inputs=1  InputSameDT=on  SaturateOnIntegerOverflow=on  OutDataTypeStr=Inherit: Same as first input
  Sum5 : Sum  Inputs=+-  InputSameDT=on  SaturateOnIntegerOverflow=on  OutDataTypeStr=Inherit: Same as first input
  Sum6 : Sum  Inputs=+-  InputSameDT=on  SaturateOnIntegerOverflow=on  OutDataTypeStr=Inherit: Same as first input
  pu->V : Gain  Gain=1/sqrt(3)  SaturateOnIntegerOverflow=on  OutDataTypeStr=Inherit: Same as input  ParamDataTypeStr=Inherit: Same as input
  pu->V1 : Gain  Gain=1/3  SaturateOnIntegerOverflow=on  OutDataTypeStr=Inherit: Same as input  ParamDataTypeStr=Inherit: Same as input
  pu->V2 : Gain  Gain=1/3  SaturateOnIntegerOverflow=on  OutDataTypeStr=Inherit: Same as input  ParamDataTypeStr=Inherit: Same as input
  P : Outport  VectorParamsAs1DForOutWhenUnconnected=off
  Q : Outport  Port=2  VectorParamsAs1DForOutWhenUnconnected=off
  wires:
  pu->V2/1 -> Q/1
  pu->V1/1 -> P/1
  Sum1/1 -> pu->V/1
  Product3/1 -> Sum1/1
  Product1/1 -> Sum4/1
  v_abc_pu/1 -> Product1/1, Demux/1
  i_abc_pu/1 -> Product1/2, Product3/2
  Sum4/1 -> pu->V1/1
  Demux/1 -> Sum/1, Sum6/2
  Demux/2 -> Sum/2, Sum5/1
  Demux/3 -> Sum5/2, Sum6/1
  Sum/1 -> Mux/3
  Sum5/1 -> Mux/1
  Sum6/1 -> Mux/2
  Mux/1 -> Product3/1
  pu->V/1 -> pu->V2/1  "Q"

== system Sim3_GFo_L_Filter/VSC_pwm/Control loops/Current Limitation ==
  note: Current limitation
  Vm_dq* : Inport
  Ig_dq : Inport  Port=2
  vg_dq : Inport  Port=3
  Constant : Constant  Value=I_max_pu
  Current control : Subsystem
  Demux : Demux  Outputs=2
  Demux2 : Demux  Outputs=2
  Inverse Current control : Subsystem
  Mux : Mux  Inputs=2
  Product{,1..3} (4 alike) : Product
  Saturation Dynamic : simulink/Discontinuities/Saturation Dynamic  OutMin=[]  OutMax=[]  OutDataTypeStr=Inherit: Same as second input  OutDataType=fixdt(1, 16)  OutScaling=2^-10  DoSatur=off
  Sqrt : Sqrt  SaturateOnIntegerOverflow=on
  Sum : Sum
  Trigonometric Function : Trigonometry  Operator=atan2  NumberOfIterations=5  OutputSignalType=real
  Trigonometric Function1 : Trigonometry  Operator=cos
  Trigonometric Function2 : Trigonometry
  w_set1 : Constant
  w_set2 : Constant
  w_set3 : Constant  Value=0
  Vm_dq_sat : Outport  VectorParamsAs1DForOutWhenUnconnected=off
  wires:
  w_set3/1 -> Saturation Dynamic/3
  Constant/1 -> Saturation Dynamic/1
  Mux/1 -> Current control/1(Ig_dq0*)
  Product/1 -> Mux/1
  Demux/1 -> Product1/1, Product1/2
  Demux/2 -> Product2/1, Product2/2
  Trigonometric Function2/1 -> Product3/2
  Product2/1 -> Sum/2
  Trigonometric Function1/1 -> Product/2
  Demux2/1 -> Trigonometric Function/2
  Trigonometric Function/1 -> Trigonometric Function2/1, Trigonometric Function1/1
  Saturation Dynamic/1 -> Product/1, Product3/1
  Product1/1 -> Sum/1
  Sqrt/1 -> Saturation Dynamic/2
  Demux2/2 -> Trigonometric Function/1
  Inverse Current control/1(Is_dq*) -> Demux2/1, Demux/1
  Sum/1 -> Sqrt/1
  Product3/1 -> Mux/2
  Ig_dq/1 -> Inverse Current control/2(Ig_dq), Current control/2(Ig_dq0)
  w_set1/1 -> Inverse Current control/4(w)
  w_set2/1 -> Current control/4(w)
  vg_dq/1 -> Current control/3(vg_dq0), Inverse Current control/3(vg_dq)
  Vm_dq*/1 -> Inverse Current control/1(Vm_dq*)
  Current control/1(vm) -> Vm_dq_sat/1

== system Sim3_GFo_L_Filter/VSC_pwm/Control loops/Power Control Loops ==
  P_mes : Inport
  P_set : Inport  Port=2
  delta_PLL : Inport  Port=3
  w_PLL : Inport  Port=4
  Compare To Constant : simulink/Logic and Bit Operations/Compare To Constant  relop===  const=1  OutDataTypeStr=boolean
  Compare To Constant1 : simulink/Logic and Bit Operations/Compare To Constant  relop===  const=2  OutDataTypeStr=boolean
  Compare To Constant2 : simulink/Logic and Bit Operations/Compare To Constant  relop===  const=3  OutDataTypeStr=boolean
  Inertia Less : Subsystem
  Multiport Switch : MultiPortSwitch
  Multiport Switch1 : MultiPortSwitch
  Mux : Mux  Inputs=[1 1]
  PI Controler : Subsystem
  Trigonometric Function : Trigonometry  Operator=cos
  Trigonometric Function1 : Trigonometry
  VSM : Subsystem
  w_set{1..4} (4 alike) : Constant  Value=Chosen_Strategy
  w_set_pu : Constant
  f : Outport  PortDimensions=1  VectorParamsAs1DForOutWhenUnconnected=off
  Theta : Outport  Port=2  VectorParamsAs1DForOutWhenUnconnected=off
  CosSinTheta : Outport  Port=3  PortDimensions=2  VectorParamsAs1DForOutWhenUnconnected=off
  wires:
  Multiport Switch1/1 -> Trigonometric Function1/1, Trigonometric Function/1, Theta/1
  Trigonometric Function1/1 -> Mux/2
  Mux/1 -> CosSinTheta/1
  Trigonometric Function/1 -> Mux/1
  Compare To Constant2/1 -> PI Controler/Enable
  Compare To Constant1/1 -> VSM/Enable
  Compare To Constant/1 -> Inertia Less/Enable
  w_set4/1 -> Compare To Constant2/1
  w_set2/1 -> Compare To Constant1/1
  w_set3/1 -> Compare To Constant/1
  Inertia Less/1(frequency) -> Multiport Switch/2
  Multiport Switch/1 -> f/1
  Inertia Less/2(theta) -> Multiport Switch1/2
  VSM/2(theta) -> Multiport Switch1/3
  w_set1/1 -> Multiport Switch/1, Multiport Switch1/1
  VSM/1(frequency) -> Multiport Switch/3
  PI Controler/1(frequency) -> Multiport Switch/4
  PI Controler/2(theta) -> Multiport Switch1/4
  w_set_pu/1 -> PI Controler/3(w_set_pu)
  w_PLL/1 -> Inertia Less/4(w_PLL), VSM/3(w_PLL)
  delta_PLL/1 -> Inertia Less/3(delta_PLL)
  P_set/1 -> Inertia Less/2(P_set), VSM/2(P_set), PI Controler/2(P_set)
  P_mes/1 -> Inertia Less/1(P_mes), VSM/1(P_mes), PI Controler/1(P_mes)

== system Sim3_GFo_L_Filter/VSC_pwm/Control loops/Transient Damping Resistance ==
  ig_dq : Inport
  Filter w_LF : Subsystem
      mask Display: disp('\omega_{LF} / (s + \omega_{LF})','texmode','on')
  Sum5 : Sum  Inputs=|+-
  nq1 : Gain  Gain=Rv
  "Delta_E_dq " : Outport  VectorParamsAs1DForOutWhenUnconnected=off
  wires:
  nq1/1 -> Filter w_LF/1(e), Sum5/2
  Filter w_LF/1(s) -> Sum5/1
  Sum5/1 -> "Delta_E_dq "/1
  ig_dq/1 -> nq1/1

== system Sim3_GFo_L_Filter/VSC_pwm/Control loops/VI ==
  note: VI triggering and threshold computation
  note: VI
  i_VI_dq : Inport
  Demux1 : Demux  Outputs=2
      settings: DisplayOption=none
  Gain5 : Gain  Gain=DX_DR
  Gain6 : Gain  Gain=Kp_Rvi_pu
  Gain9 : Gain  Gain=DX_DR
  I_thresh : Constant  Value=I_thresh_pu
  Mux2 : Mux  Inputs=2
  Saturation : Saturate  UpperLimit=inf  LowerLimit=0
  Sum1 : Sum  Inputs=-+|
  Sum7 : Sum  Inputs=|+-
  Sum8 : Sum  Inputs=++|
  dq to phasor : Subsystem
  product{,1..3} (4 alike) : Product  InputSameDT=on  RndMeth=Zero  SaturateOnIntegerOverflow=on  OutDataTypeStr=Inherit: Same as first input
  I_rms : Outport  VectorParamsAs1DForOutWhenUnconnected=off
  Delta_E_dq : Outport  Port=2  VectorParamsAs1DForOutWhenUnconnected=off
  wires:
  Sum1/1 -> Saturation/1
  dq to phasor/1(rms) -> Sum1/2, I_rms/1  "I_rms"
  Saturation/1 -> Gain6/1
  I_thresh/1 -> Sum1/1
  Mux2/1 -> Delta_E_dq/1
  Gain6/1 -> product3/2, product/1, product1/2, product2/2
  product3/1 -> Gain5/1
  product/1 -> Gain9/1
  Demux1/1 -> product1/1, product/2  "igd"
  Demux1/2 -> product2/1, product3/1  "igq"
  product1/1 -> Sum7/1
  Gain5/1 -> Sum7/2
  Gain9/1 -> Sum8/1
  product2/1 -> Sum8/2
  Sum7/1 -> Mux2/1
  Sum8/1 -> Mux2/2
  i_VI_dq/1 -> dq to phasor/1(dq_mes), Demux1/1

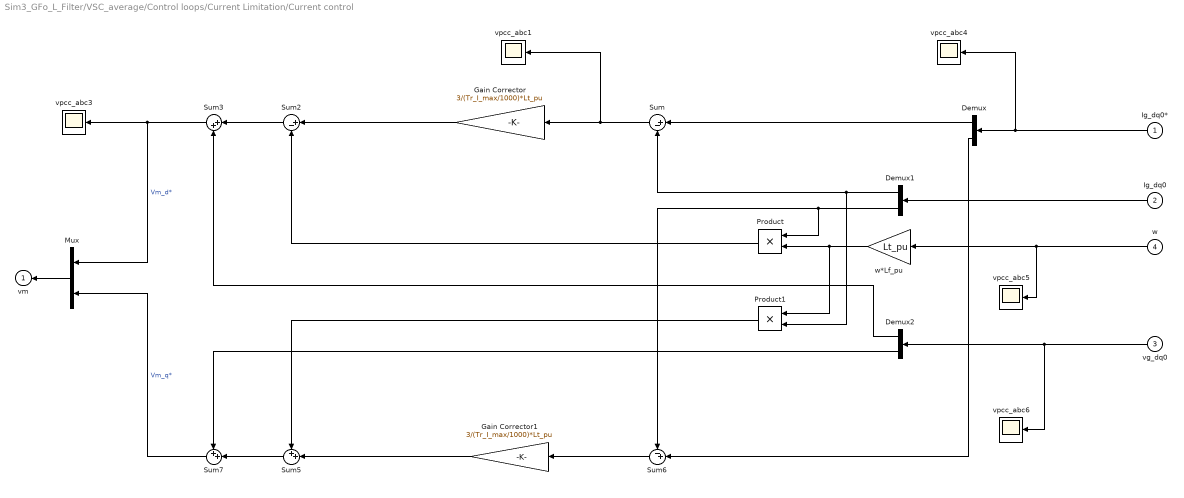
== system Sim3_GFo_L_Filter/VSC_average/Control loops/Current Limitation/Current control ==
  Ig_dq0* : Inport
  Ig_dq0 : Inport  Port=2
  vg_dq0 : Inport  Port=3
  w : Inport  Port=4
  Demux : Demux  Outputs=2
  Demux1 : Demux  Outputs=2
  Demux2 : Demux  Outputs=2
  Gain Corrector : Gain  Gain=3/(Tr_I_max/1000)*Lt_pu
  Gain Corrector1 : Gain  Gain=3/(Tr_I_max/1000)*Lt_pu
  Mux : Mux  Inputs=2
  Product : Product  RndMeth=Zero
  Product1 : Product  RndMeth=Zero
  Sum : Sum  Inputs=|+-
  Sum2 : Sum  Inputs=|+-
  Sum3 : Sum  Inputs=|++
  Sum5 : Sum  Inputs=++|
  Sum6 : Sum  Inputs=-+|
  Sum7 : Sum  Inputs=++|
  vpcc_abc{1,3..6} (5 alike) : Scope
  w*Lf_pu : Gain  Gain=Lt_pu
  vm : Outport  InitialOutput=0  VectorParamsAs1DForOutWhenUnconnected=off
  wires:
  Demux2/2 -> Sum7/1
  Demux2/1 -> Sum3/2
  w/1 -> vpcc_abc5/1, w*Lf_pu/1
  Sum/1 -> vpcc_abc1/1, Gain Corrector/1
  Sum7/1 -> Mux/2  "Vm_q*"
  Sum3/1 -> Mux/1, vpcc_abc3/1  "Vm_d*"
  Sum5/1 -> Sum7/2
  Product1/1 -> Sum5/1
  Gain Corrector1/1 -> Sum5/2
  Demux/2 -> Sum6/2
  Sum2/1 -> Sum3/1
  Product/1 -> Sum2/2
  Demux1/2 -> Sum6/1, Product/1
  w*Lf_pu/1 -> Product/2, Product1/1
  Gain Corrector/1 -> Sum2/1
  Demux1/1 -> Sum/2, Product1/2
  Demux/1 -> Sum/1
  Ig_dq0/1 -> Demux1/1
  vg_dq0/1 -> Demux2/1, vpcc_abc6/1
  Sum6/1 -> Gain Corrector1/1
  Ig_dq0*/1 -> vpcc_abc4/1, Demux/1
  Mux/1 -> vm/1

== system Sim3_GFo_L_Filter/VSC_average/Control loops/Current Limitation/Inverse Current control ==
  Vm_dq* : Inport
  Ig_dq : Inport  Port=2
  vg_dq : Inport  Port=3
  w : Inport  Port=4
  Demux : Demux  Outputs=2
  Demux1 : Demux  Outputs=2
  Demux2 : Demux  Outputs=2
  Gain Corrector2 : Gain  Gain=1/(3/(Tr_I_max/1000)*Lt_pu)
  Gain Corrector3 : Gain  Gain=1/(3/(Tr_I_max/1000)*Lt_pu)
  Mux : Mux  Inputs=2
  Product : Product  RndMeth=Zero
  Product1 : Product  RndMeth=Zero
  Sum : Sum  Inputs=|+-
  Sum2 : Sum  Inputs=|++
  Sum3 : Sum  Inputs=|++
  Sum5 : Sum  Inputs=-+|
  Sum6 : Sum  Inputs=-+|
  Sum7 : Sum  Inputs=++|
  w*Lf_pu : Gain  Gain=Lt_pu
  Is_dq* : Outport  InitialOutput=0  VectorParamsAs1DForOutWhenUnconnected=off
  wires:
  vg_dq/1 -> Demux2/1
  Ig_dq/1 -> Demux1/1
  Vm_dq*/1 -> Demux/1
  Demux/1 -> Sum/1
  Demux1/1 -> Sum3/2, Product1/2
  Sum/1 -> Sum2/1
  w*Lf_pu/1 -> Product1/1, Product/2
  Product/1 -> Sum2/2
  Sum2/1 -> Gain Corrector3/1
  Mux/1 -> Is_dq*/1
  Demux/2 -> Sum6/2
  Sum6/1 -> Sum5/2
  Sum5/1 -> Gain Corrector2/1
  Sum3/1 -> Mux/1  "is_d*"
  Sum7/1 -> Mux/2  "is_q*"
  w/1 -> w*Lf_pu/1
  Demux1/2 -> Sum7/1, Product/1
  Gain Corrector3/1 -> Sum3/1
  Demux2/1 -> Sum/2
  Demux2/2 -> Sum6/1
  Product1/1 -> Sum5/1
  Gain Corrector2/1 -> Sum7/2

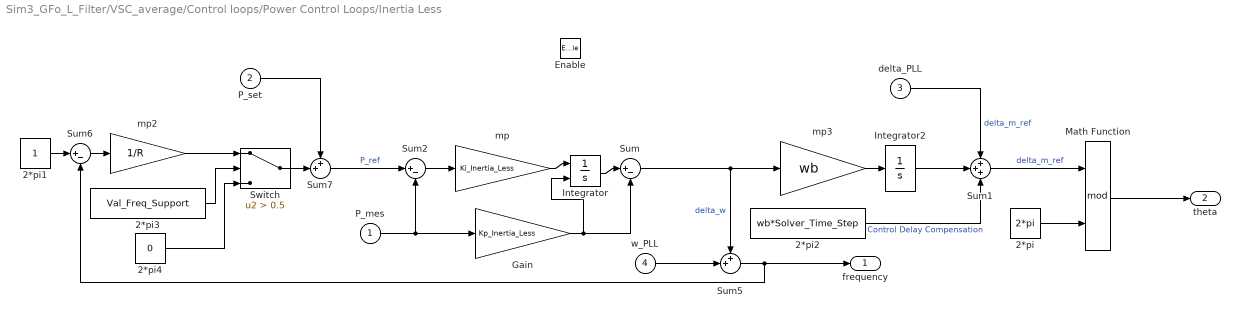
== system Sim3_GFo_L_Filter/VSC_average/Control loops/Power Control Loops/Inertia Less ==
  P_mes : Inport
  P_set : Inport  Port=2
  delta_PLL : Inport  Port=3
  w_PLL : Inport  Port=4
  Enable : EnablePort
  2*pi : Constant  Value=2*pi
  2*pi1 : Constant
  2*pi2 : Constant  Value=wb*Solver_Time_Step
  2*pi3 : Constant  Value=Val_Freq_Support
  2*pi4 : Constant  Value=0
  Gain : Gain  Gain=Kp_Inertia_Less
  Integrator : Integrator  InitialConditionSource=external
  Integrator2 : Integrator  InitialCondition=(Theta_vsc0)*pi/180-Theta0*pi/180
  Math Function : Math  Operator=mod  SaturateOnIntegerOverflow=on
  Sum : Sum  Inputs=|+-
  Sum1 : Sum  Inputs=+++
  Sum2 : Sum  Inputs=|+-
  Sum5 : Sum  Inputs=++|
  Sum6 : Sum  Inputs=|+-
  Sum7 : Sum  Inputs=++|
  Switch : Switch  Criteria=u2 > Threshold  Threshold=0.5
  mp : Gain  Gain=Ki_Inertia_Less
  mp2 : Gain  Gain=1/R
  mp3 : Gain  Gain=wb
  frequency : Outport  VectorParamsAs1DForOutWhenUnconnected=off
  theta : Outport  Port=2  VectorParamsAs1DForOutWhenUnconnected=off
  wires:
  Gain/1 -> Sum/2, Integrator/2
  Integrator/1 -> Sum/1
  2*pi4/1 -> Switch/3
  2*pi3/1 -> Switch/2
  mp2/1 -> Switch/1
  Integrator2/1 -> Sum1/2
  2*pi2/1 -> Sum1/3  "Control Delay Compensation"
  Sum5/1 -> Sum6/2, frequency/1
  w_PLL/1 -> Sum5/2
  delta_PLL/1 -> Sum1/1  "delta_m_ref"
  mp/1 -> Integrator/1
  mp3/1 -> Integrator2/1
  Sum/1 -> Sum5/1, mp3/1  "delta_w"
  Math Function/1 -> theta/1
  Switch/1 -> Sum7/2
  P_mes/1 -> Sum2/2, Gain/1
  Sum7/1 -> Sum2/1  "P_ref"
  P_set/1 -> Sum7/1
  Sum6/1 -> mp2/1
  2*pi1/1 -> Sum6/1
  2*pi/1 -> Math Function/2
  Sum1/1 -> Math Function/1  "delta_m_ref"
  Sum2/1 -> mp/1

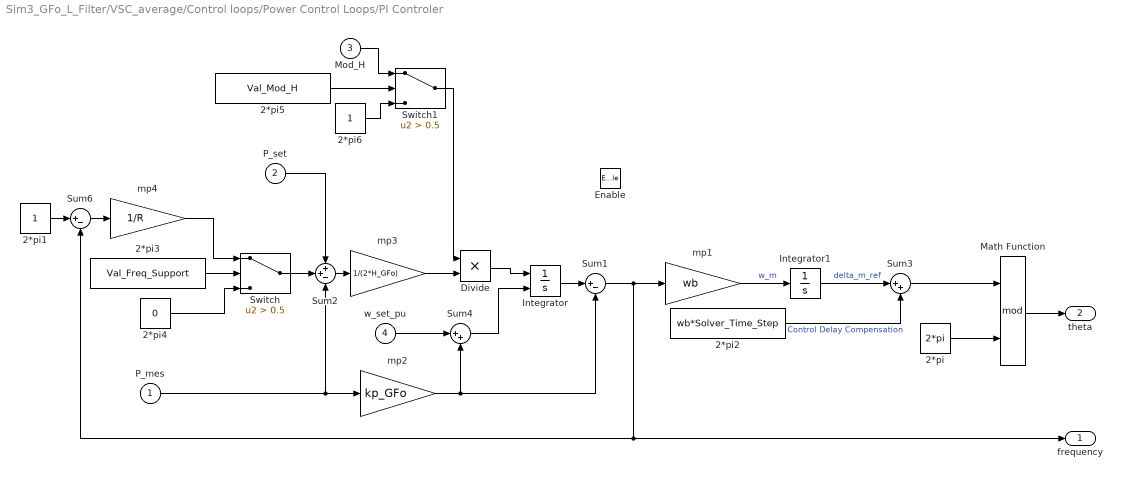
== system Sim3_GFo_L_Filter/VSC_average/Control loops/Power Control Loops/PI Controler ==
  P_mes : Inport
  P_set : Inport  Port=2
  Mod_H : Inport  Port=3
  w_set_pu : Inport  Port=4
  Enable : EnablePort
  2*pi : Constant  Value=2*pi
  2*pi1 : Constant
  2*pi2 : Constant  Value=wb*Solver_Time_Step
  2*pi3 : Constant  Value=Val_Freq_Support
  2*pi4 : Constant  Value=0
  2*pi5 : Constant  Value=Val_Mod_H
  2*pi6 : Constant
  Divide : Product  Inputs=**
  Integrator : Integrator  InitialConditionSource=external
  Integrator1 : Integrator  InitialCondition=(Theta_vsc0)*pi/180
  Math Function : Math  Operator=mod  SaturateOnIntegerOverflow=on
  Sum1 : Sum  Inputs=|+-
  Sum2 : Sum  Inputs=++-
  Sum3 : Sum  Inputs=|++
  Sum4 : Sum  Inputs=|++
  Sum6 : Sum  Inputs=|+-
  Switch : Switch  Criteria=u2 > Threshold  Threshold=0.5
  Switch1 : Switch  Criteria=u2 > Threshold  Threshold=0.5
  mp1 : Gain  Gain=wb
  mp2 : Gain  Gain=kp_GFo
  mp3 : Gain  Gain=1/(2*H_GFo)
  mp4 : Gain  Gain=1/R
  frequency : Outport  VectorParamsAs1DForOutWhenUnconnected=off
  theta : Outport  Port=2  VectorParamsAs1DForOutWhenUnconnected=off
  wires:
  Switch1/1 -> Divide/1
  Divide/1 -> Integrator/1
  Mod_H/1 -> Switch1/1
  2*pi6/1 -> Switch1/3
  2*pi5/1 -> Switch1/2
  Switch/1 -> Sum2/2
  2*pi4/1 -> Switch/3
  Sum6/1 -> mp4/1
  2*pi3/1 -> Switch/2
  2*pi1/1 -> Sum6/1
  mp4/1 -> Switch/1
  Sum4/1 -> Integrator/2
  mp3/1 -> Divide/2
  mp2/1 -> Sum4/2, Sum1/2
  P_mes/1 -> mp2/1, Sum2/3
  2*pi2/1 -> Sum3/2  "Control Delay Compensation"
  Sum3/1 -> Math Function/1
  mp1/1 -> Integrator1/1  "w_m"
  Sum1/1 -> Sum6/2, frequency/1, mp1/1
  Integrator/1 -> Sum1/1
  P_set/1 -> Sum2/1
  w_set_pu/1 -> Sum4/1
  2*pi/1 -> Math Function/2
  Math Function/1 -> theta/1
  Integrator1/1 -> Sum3/1  "delta_m_ref"
  Sum2/1 -> mp3/1

== system Sim3_GFo_L_Filter/VSC_average/Control loops/Power Control Loops/Subsystem ==
  Delta_E_dq : Inport
  Constant : Constant
  Constant1 : Constant  Value=2
  Delay : Delay  DelayLength=1  InitialCondition=1
  Demux : Demux  Outputs=2
  Pow : Math  Operator=pow  RndMeth=Zero  SaturateOnIntegerOverflow=on
  Square : Math  Operator=square  RndMeth=Zero  SaturateOnIntegerOverflow=on
  Square1 : Math  Operator=square  RndMeth=Zero  SaturateOnIntegerOverflow=on
  Sum : Sum  Inputs=|+-
  Sum5 : Sum
  Mod_h : Outport  VectorParamsAs1DForOutWhenUnconnected=off
  wires:
  Delay/1 -> Demux/1
  Sum/1 -> Square/1
  Demux/1 -> Sum/2
  Square1/1 -> Sum5/2
  Sum5/1 -> Pow/1
  Constant/1 -> Sum/1
  Demux/2 -> Square1/1
  Constant1/1 -> Pow/2
  Pow/1 -> Mod_h/1
  Square/1 -> Sum5/1
  Delta_E_dq/1 -> Delay/1
